simulink model "ROS_SIMULINK_Concept_Testing_ABB_6DOF"  (R2023a)
settings: Solver=FixedStepDiscrete  StartTime=0.0  StopTime=inf  FixedStep=0.004  RelTol=1e-3
model workspace (MAT data in the model file):
  SL_ROS_VariableLengthArrays_MaxSizes.CommonInfo.ArrayTruncateAction = 'EmitWarning'
  SL_ROS_VariableLengthArrays_MaxSizes.MsgTypeMap = containers.Map
  SL_ROS_VariableLengthArrays_MaxSizes.MsgTypeMap.serialization.keys = {'std_msgs/Float64MultiArray'}
  SL_ROS_VariableLengthArrays_MaxSizes.MsgTypeMap.serialization.values{1}.PropertyName = 'Data'
  SL_ROS_VariableLengthArrays_MaxSizes.MsgTypeMap.serialization.values{1}.DataType = 'double'
  SL_ROS_VariableLengthArrays_MaxSizes.MsgTypeMap.serialization.values{1}.MaxLength = 6
  SL_ROS_VariableLengthArrays_MaxSizes.MsgTypeMap.serialization.uniformity = 0
  SL_ROS_VariableLengthArrays_MaxSizes.MsgTypeMap.serialization.keyType = 'char'
  SL_ROS_VariableLengthArrays_MaxSizes.MsgTypeMap.serialization.valueType = 'any'
undefined symbols (not defined in the file): Data, Data_SL_Info
libraries: slpidlib x6, robotlib x3, simulink x3, eeGeneralControl x2, simulink_extras x1
settings Model: Creator=LYA31  LastModifiedBy=LYA31
settings OptimizationCC: EnhancedBackFolding=on  PassReuseOutputArgsAs=Individual arguments  ZeroExternalMemoryAtStartup=off  ZeroInternalMemoryAtStartup=off  MaxStackSize=64  OptimizeBlockOrder=speed  DifferentSizesBufferReuse=on  EfficientTunableParamExpr=on
settings DebuggingCC: ParameterTunabilityLossMsg=error
settings HardwareCC: ProdBitPerPointer=32  ProdBitPerSizeT=32  ProdBitPerPtrDiffT=32  ProdLargestAtomicFloat=None  ProdIntDivRoundTo=Undefined  ProdEndianess=Unspecified  ProdWordSize=32  ProdHWDeviceType=Generic->Unspecified (assume 32-bit Generic)
settings SFSimCC: MATLABDynamicMemAlloc=off
settings RTWCC: Description=Embedded Coder  SystemTargetFile=ert.tlc  HardwareBoard=Robot Operating System (ROS)  TLCOptions="-aInlineSetEventsForThisBaseRateFcn=TLC_FALSE -aSuppressMultiTaskScheduler=TLC_FALSE  -aRateBasedStepFcn=0"  TemplateMakefile=ert_default_tmf  Toolchain=Catkin  TargetLang=C++
settings CodeAppCC: ForceParamTrailComments=on  IgnoreCustomStorageClasses=off  OperatorAnnotations=on  SimulinkDataObjDesc=on  SFDataObjDesc=on  InsertBlockDesc=on

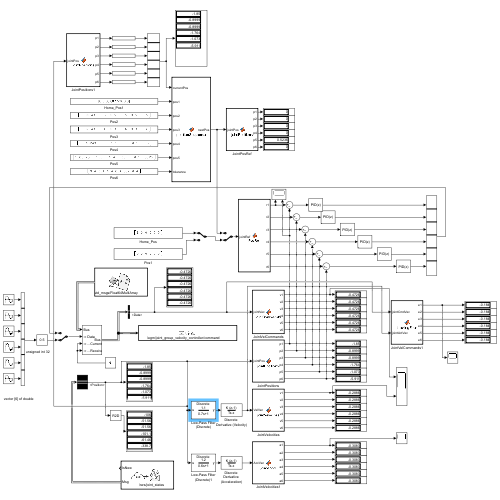
[thumbnail: Simulink's stored preview of the top-level diagram]
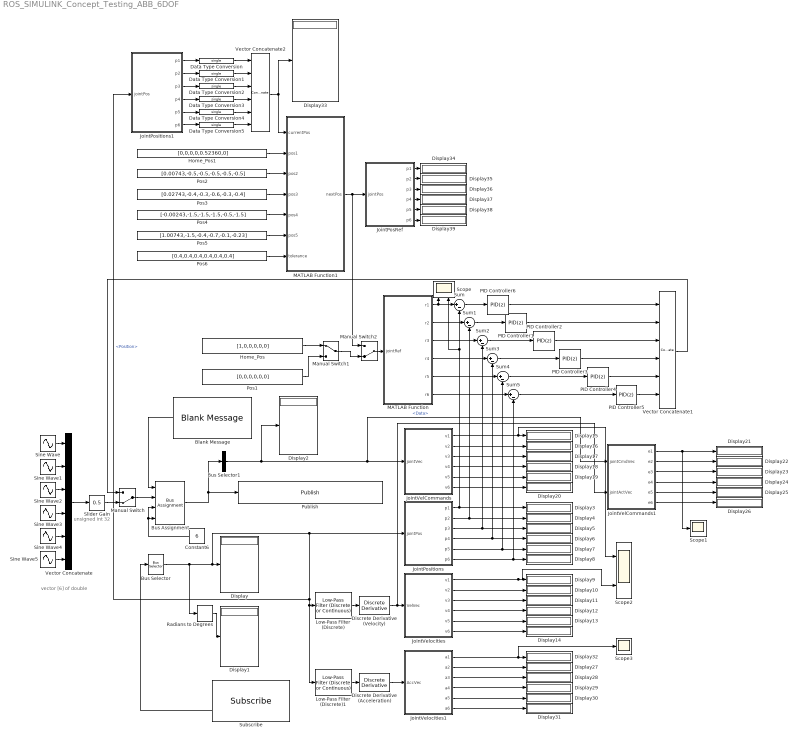
== system ROS_SIMULINK_Concept_Testing_ABB_6DOF ==
  note: unsigned int 32
  note: vector [6] of double
  Blank Message : robotlib/Blank Message  messageClass=Message  entityType=std_msgs/Float64MultiArray  messageType=std_msgs/Float64MultiArray  SampleTime=inf  legacyBusStruct=off
  Bus Assignment : BusAssignment  AssignedSignals=Data,Data_SL_Info.CurrentLength,Data_SL_Info.ReceivedLength
  Bus Selector : BusSelector  OutputSignals=Position
  Bus Selector1 : BusSelector  OutputSignals=Data
  Constant6 : Constant  Value=6  OutDataTypeStr=uint32  SampleTime=0.004
  Data Type Conversion{,1..5} (6 alike) : DataTypeConversion  OutDataTypeStr=single  SaturateOnIntegerOverflow=off  RndMeth=Floor
  Discrete Derivative (Acceleration) : simulink/Discrete/Discrete Derivative  gainval=1.0  ICPrevScaledInput=0.0  OutMin=[]  OutMax=[]  OutDataTypeStr=double  OutputDataTypeScalingMode=double  OutDataType=fixdt(1, 16)  OutScaling=2^-10  DoSatur=off
  Discrete Derivative (Velocity) : simulink/Discrete/Discrete Derivative  gainval=1.0  ICPrevScaledInput=0.0  OutMin=[]  OutMax=[]  OutDataTypeStr=double  OutputDataTypeScalingMode=double  OutDataType=fixdt(1, 16)  OutScaling=2^-10  DoSatur=off
  Display{,1..39} (40 alike) : Display
  Home_Pos : Constant  Value=[1,0,0,0,0,0]
  Home_Pos1 : Constant  Value=[0,0,0,0,0.52360,0]  OutDataTypeStr=double
  JointPosRef : MATLAB Function  TreatAsAtomicUnit=on
  JointPositions : MATLAB Function  TreatAsAtomicUnit=on
  JointPositions1 : MATLAB Function  TreatAsAtomicUnit=on
  JointVelCommands : MATLAB Function  TreatAsAtomicUnit=on
  JointVelCommands1 : MATLAB Function  TreatAsAtomicUnit=on
  JointVelocities : MATLAB Function  TreatAsAtomicUnit=on
  JointVelocities1 : MATLAB Function  TreatAsAtomicUnit=on
  Low-Pass Filter (Discrete) : eeGeneralControl/Low-Pass Filter (Discrete or Continuous)  K=1.1  T=0.7  B=inf  A=-inf  init_option=Inherited from block input  x0=0  Ts=-1
  Low-Pass Filter (Discrete)1 : eeGeneralControl/Low-Pass Filter (Discrete or Continuous)  K=1.2  T=0.6  B=inf  A=-inf  init_option=Inherited from block input  x0=0  Ts=-1
  MATLAB Function : MATLAB Function  TreatAsAtomicUnit=on
  MATLAB Function1 : MATLAB Function  TreatAsAtomicUnit=on
  Manual Switch : ManualSwitch  CurrentSetting=0
  Manual Switch1 : ManualSwitch
  Manual Switch2 : ManualSwitch  CurrentSetting=0
  PID Controller{1..5} (5 alike) : slpidlib/PID Controller  Controller=PID  Form=Ideal  TimeDomain=Discrete-time  UseExternalTs=off  SampleTime=-1  IntegratorMethod=Forward Euler  FilterMethod=Forward Euler  ControllerParametersSource=internal  P=2.4  I=0.01  UseKiTs=off  D=0.7  N=100  UseFilter=on  TunerSelectOption=Transfer Function Based (PID Tuner App)  InitialConditionSource=internal  InitialConditionForIntegrator=0  InitialConditionForFilter=0  DifferentiatorICPrevScaledInput=0  ExternalReset=none  TrackingMode=off  Kt=1  LimitOutput=off  SatLimitsSource=internal  UpperSaturationLimit=inf  LowerSaturationLimit=-inf  LinearizeAsGain=on  AntiWindupMode=none  Kb=1  LimitIntegrator=off  UpperIntegratorSaturationLimit=inf  LowerIntegratorSaturationLimit=-inf  POutMin=[]  POutMax=[]  IOutMin=[]  IOutMax=[]  DOutMin=[]  DOutMax=[]  NOutMin=[]  NOutMax=[]  SumOutMin=[]  SumOutMax=[]  SaturationOutMin=[]  SaturationOutMax=[]  PParamMin=[]  PParamMax=[]  IParamMin=[]  IParamMax=[]  DParamMin=[]  DParamMax=[]  NParamMin=[]  NParamMax=[]  KbParamMin=[]  KbParamMax=[]  KtParamMin=[]  KtParamMax=[]  KbOutMin=[]  KbOutMax=[]  KtOutMin=[]  KtOutMax=[]  IntegratorOutMin=[]  IntegratorOutMax=[]  FilterOutMin=[]  FilterOutMax=[]  SumI1OutMin=[]  SumI1OutMax=[]  SumI2OutMin=[]  SumI2OutMax=[]  SumI3OutMin=[]  SumI3OutMax=[]  SumI4OutMin=[]  SumI4OutMax=[]  SumDOutMin=[]  SumDOutMax=[]  DifferentiatorOutMin=[]  DifferentiatorOutMax=[]  FilterDiffOutCoefMin=[]  FilterDiffOutCoefMax=[]  ReciprocalOutMin=[]  ReciprocalOutMax=[]  SumDenOutMin=[]  SumDenOutMax=[]  SumNumOutMin=[]  SumNumOutMax=[]  DivideOutMin=[]  DivideOutMax=[]  UdiffTsProdOutMin=[]  UdiffTsProdOutMax=[]  NTsProdOutMin=[]  NTsProdOutMax=[]  UintegralTsProdOutMin=[]  UintegralTsProdOutMax=[]  UngainTsProdOutMin=[]  UngainTsProdOutMax=[]  ClampingZeroOutDataTypeStr=Inherit: Inherit via back propagation  ClampingZeroOutMin=[]  ClampingZeroOutMax=[]  FilterDenConstantOutDataTypeStr=Inherit: Inherit via back propagation  FilterDenConstantOutMin=[]  FilterDenConstantOutMax=[]  PCopyOutDataTypeStr=Inherit: Inherit via back propagation  PCopyOutMin=[]  PCopyOutMax=[]  NCopyOutDataTypeStr=Inherit: Inherit via back propagation  NCopyOutMin=[]  NCopyOutMax=[]  IntegratorContinuousStateAttributes=''  IntegratorStateMustResolveToSignalObject=off  IntegratorRTWStateStorageClass=Auto  FilterContinuousStateAttributes=''  FilterStateMustResolveToSignalObject=off  FilterRTWStateStorageClass=Auto  ParallelPVariant=Passthrough  IdealPVariant=InternalParameters  IVariant=InternalParameters  DVariant=InternalParameters  IntegratorVariant=Discrete  SatVariant=Disabled  AWVariant=Passthrough  PCopyVariant=Disabled  TRVariant=Disabled  FdbkBlocksVariant=Forward  IdealPFdbkVariant=Disabled  SatFdbkVariant=Disabled  DerivativeFilterVariant=ForwardEulerFilter  NVariant=InternalParameters  NCopyVariant=Disabled  FilterICVariant=InternalICsFilter  IntegratorICVariant=InternalICs  ExternalResetVariant=Disabled  TRSumVariant=Passthrough  SumFdbkVariant=Disabled  SumVariant=Sum_PID  TsampFilterVariant=InternalTs  TsampNgainVariant=Passthrough  TsampIntegralVariant=Disabled_SignalSpec  ExternalSaturationOutDataTypeStr=Inherit: Same as second input
  PID Controller6 : slpidlib/PID Controller  Controller=PID  Form=Ideal  TimeDomain=Discrete-time  UseExternalTs=off  SampleTime=-1  IntegratorMethod=Forward Euler  FilterMethod=Forward Euler  ControllerParametersSource=internal  P=9  I=0  UseKiTs=off  D=0  N=100  UseFilter=on  TunerSelectOption=Transfer Function Based (PID Tuner App)  InitialConditionSource=internal  InitialConditionForIntegrator=0  InitialConditionForFilter=0  DifferentiatorICPrevScaledInput=0  ExternalReset=none  TrackingMode=off  Kt=1  LimitOutput=off  SatLimitsSource=internal  UpperSaturationLimit=inf  LowerSaturationLimit=-inf  LinearizeAsGain=on  AntiWindupMode=none  Kb=1  LimitIntegrator=off  UpperIntegratorSaturationLimit=inf  LowerIntegratorSaturationLimit=-inf  POutMin=[]  POutMax=[]  IOutMin=[]  IOutMax=[]  DOutMin=[]  DOutMax=[]  NOutMin=[]  NOutMax=[]  SumOutMin=[]  SumOutMax=[]  SaturationOutMin=[]  SaturationOutMax=[]  PParamMin=[]  PParamMax=[]  IParamMin=[]  IParamMax=[]  DParamMin=[]  DParamMax=[]  NParamMin=[]  NParamMax=[]  KbParamMin=[]  KbParamMax=[]  KtParamMin=[]  KtParamMax=[]  KbOutMin=[]  KbOutMax=[]  KtOutMin=[]  KtOutMax=[]  IntegratorOutMin=[]  IntegratorOutMax=[]  FilterOutMin=[]  FilterOutMax=[]  SumI1OutMin=[]  SumI1OutMax=[]  SumI2OutMin=[]  SumI2OutMax=[]  SumI3OutMin=[]  SumI3OutMax=[]  SumI4OutMin=[]  SumI4OutMax=[]  SumDOutMin=[]  SumDOutMax=[]  DifferentiatorOutMin=[]  DifferentiatorOutMax=[]  FilterDiffOutCoefMin=[]  FilterDiffOutCoefMax=[]  ReciprocalOutMin=[]  ReciprocalOutMax=[]  SumDenOutMin=[]  SumDenOutMax=[]  SumNumOutMin=[]  SumNumOutMax=[]  DivideOutMin=[]  DivideOutMax=[]  UdiffTsProdOutMin=[]  UdiffTsProdOutMax=[]  NTsProdOutMin=[]  NTsProdOutMax=[]  UintegralTsProdOutMin=[]  UintegralTsProdOutMax=[]  UngainTsProdOutMin=[]  UngainTsProdOutMax=[]  ClampingZeroOutDataTypeStr=Inherit: Inherit via back propagation  ClampingZeroOutMin=[]  ClampingZeroOutMax=[]  FilterDenConstantOutDataTypeStr=Inherit: Inherit via back propagation  FilterDenConstantOutMin=[]  FilterDenConstantOutMax=[]  PCopyOutDataTypeStr=Inherit: Inherit via back propagation  PCopyOutMin=[]  PCopyOutMax=[]  NCopyOutDataTypeStr=Inherit: Inherit via back propagation  NCopyOutMin=[]  NCopyOutMax=[]  IntegratorContinuousStateAttributes=''  IntegratorStateMustResolveToSignalObject=off  IntegratorRTWStateStorageClass=Auto  FilterContinuousStateAttributes=''  FilterStateMustResolveToSignalObject=off  FilterRTWStateStorageClass=Auto  ParallelPVariant=Passthrough  IdealPVariant=InternalParameters  IVariant=InternalParameters  DVariant=InternalParameters  IntegratorVariant=Discrete  SatVariant=Disabled  AWVariant=Passthrough  PCopyVariant=Disabled  TRVariant=Disabled  FdbkBlocksVariant=Forward  IdealPFdbkVariant=Disabled  SatFdbkVariant=Disabled  DerivativeFilterVariant=ForwardEulerFilter  NVariant=InternalParameters  NCopyVariant=Disabled  FilterICVariant=InternalICsFilter  IntegratorICVariant=InternalICs  ExternalResetVariant=Disabled  TRSumVariant=Passthrough  SumFdbkVariant=Disabled  SumVariant=Sum_PID  TsampFilterVariant=InternalTs  TsampNgainVariant=Passthrough  TsampIntegralVariant=Disabled_SignalSpec  ExternalSaturationOutDataTypeStr=Inherit: Same as second input
  Pos1 : Constant  Value=[0,0,0,0,0,0]
  Pos2 : Constant  Value=[0.00743,-0.5,-0.5,-0.5,-0.5,-0.5]  OutDataTypeStr=double
  Pos3 : Constant  Value=[0.02743,-0.4,-0.3,-0.6,-0.3,-0.4]  OutDataTypeStr=double
  Pos4 : Constant  Value=[-0.00243,-1.5,-1.5,-1.5,-0.5,-1.5]  OutDataTypeStr=double
  Pos5 : Constant  Value=[1.00743,-1.5,-0.4,-0.7,-0.1,-0.23]  OutDataTypeStr=double
  Pos6 : Constant  Value=[0.4,0.4,0.4,0.4,0.4,0.4]  OutDataTypeStr=double
  Publish : robotlib/Publish  topicSource=Select from ROS network  topic=/egm/joint_group_velocity_controller/command  messageType=std_msgs/Float64MultiArray  legacyBusStruct=off  messageQueueLength=1
  Radians to Degrees : simulink_extras/Transformations/Radians to Degrees
  Scope : Scope  NumInputPorts=2
  Scope1 : Scope
  Scope2 : Scope  NumInputPorts=2
  Scope3 : Scope
  Sine Wave{,1..5} (6 alike) : Sin  Frequency=0.5  SampleTime=0.004
  Slider Gain : simulink/Math Operations/Slider Gain  gain=0.5  low=-6  high=6
  Subscribe : robotlib/Subscribe  topicSource=Select from ROS network  topic=/rws/joint_states  messageType=sensor_msgs/JointState  SampleTime=-1  legacyBusStruct=off  messageQueueLength=1
  Sum{,1..5} (6 alike) : Sum  Inputs=|+-
  Vector Concatenate : Concatenate  NumInputs=6
  Vector Concatenate1 : Concatenate  NumInputs=6
  Vector Concatenate2 : Concatenate  NumInputs=6
  wires:
  Subscribe/2 -> Bus Selector/1
  Bus Selector/1 -> Radians to Degrees/1, JointPositions1/1(jointPos), Low-Pass Filter (Discrete)1/1, Low-Pass Filter (Discrete)/1, JointPositions/1(jointPos), Display/1  "<Position>"
  Radians to Degrees/1 -> Display1/1
  Bus Assignment/1 -> Publish/1, Bus Selector1/1
  Blank Message/1 -> Bus Assignment/1
  Bus Selector1/1 -> Display2/1, JointVelCommands/1(jointVec), JointVelCommands1/1(jointCmdVec)  "<Data>"
  Vector Concatenate/1 -> Slider Gain/1
  Constant6/1 -> Bus Assignment/3, Bus Assignment/4
  JointPositions/2(p2) -> Display4/1, Sum1/2
  JointPositions/3(p3) -> Display5/1, Sum2/2
  JointPositions/4(p4) -> Display6/1, Sum3/2
  JointPositions/5(p5) -> Display7/1, Sum4/2
  JointPositions/6(p6) -> Sum5/2, Display8/1
  Sine Wave/1 -> Vector Concatenate/1
  Sine Wave1/1 -> Vector Concatenate/2
  Sine Wave2/1 -> Vector Concatenate/3
  Sine Wave3/1 -> Vector Concatenate/4
  Sine Wave4/1 -> Vector Concatenate/5
  Sine Wave5/1 -> Vector Concatenate/6
  JointPositions/1(p1) -> Scope/2, Sum/2, Display3/1
  Low-Pass Filter (Discrete)/1 -> Discrete Derivative (Velocity)/1
  JointVelocities/2(v2) -> Display10/1
  JointVelocities/5(v5) -> Display13/1
  JointVelocities/1(v1) -> Scope2/2, Display9/1
  JointVelocities/6(v6) -> Display14/1
  JointVelocities/3(v3) -> Display11/1
  JointVelocities/4(v4) -> Display12/1
  JointVelCommands/2(v2) -> Display16/1
  JointVelCommands/5(v5) -> Display19/1
  JointVelCommands/1(v1) -> Scope2/1, Display15/1
  JointVelCommands/6(v6) -> Display20/1
  JointVelCommands/3(v3) -> Display17/1
  JointVelCommands/4(v4) -> Display18/1
  JointVelCommands1/5(e5) -> Display25/1
  JointVelCommands1/1(e1) -> Scope1/1, Display21/1
  JointVelCommands1/6(e6) -> Display26/1
  JointVelCommands1/2(e2) -> Display22/1
  JointVelCommands1/4(e4) -> Display24/1
  JointVelCommands1/3(e3) -> Display23/1
  Discrete Derivative (Acceleration)/1 -> JointVelocities1/1(AccVec)
  Low-Pass Filter (Discrete)1/1 -> Discrete Derivative (Acceleration)/1
  JointVelocities1/6(a6) -> Display31/1
  JointVelocities1/1(a1) -> Scope3/1, Display32/1
  JointVelocities1/3(a3) -> Display28/1
  JointVelocities1/4(a4) -> Display29/1
  JointVelocities1/5(a5) -> Display30/1
  JointVelocities1/2(a2) -> Display27/1
  Manual Switch/1 -> Bus Assignment/2
  Slider Gain/1 -> Manual Switch/2
  MATLAB Function/1(r1) -> Sum/1, Scope/1
  MATLAB Function/2(r2) -> Sum1/1
  MATLAB Function/3(r3) -> Sum2/1
  MATLAB Function/4(r4) -> Sum3/1
  MATLAB Function/5(r5) -> Sum4/1
  MATLAB Function/6(r6) -> Sum5/1
  Sum/1 -> PID Controller6/1
  Sum1/1 -> PID Controller1/1
  Sum2/1 -> PID Controller2/1
  Sum3/1 -> PID Controller3/1
  Sum4/1 -> PID Controller4/1
  Sum5/1 -> PID Controller5/1
  PID Controller6/1 -> Vector Concatenate1/1
  PID Controller1/1 -> Vector Concatenate1/2
  PID Controller2/1 -> Vector Concatenate1/3
  PID Controller3/1 -> Vector Concatenate1/4
  PID Controller4/1 -> Vector Concatenate1/5
  PID Controller5/1 -> Vector Concatenate1/6
  Vector Concatenate1/1 -> Manual Switch/1
  Home_Pos/1 -> Manual Switch1/1
  Pos1/1 -> Manual Switch1/2
  Manual Switch1/1 -> Manual Switch2/2
  Manual Switch2/1 -> MATLAB Function/1(jointRef)
  MATLAB Function1/1(nextPos) -> JointPosRef/1(jointPos), Manual Switch2/1
  Home_Pos1/1 -> MATLAB Function1/2(pos1)
  Pos2/1 -> MATLAB Function1/3(pos2)
  Pos3/1 -> MATLAB Function1/4(pos3)
  Pos4/1 -> MATLAB Function1/5(pos4)
  Pos5/1 -> MATLAB Function1/6(pos5)
  Pos6/1 -> MATLAB Function1/7(tolerance)
  JointPositions1/1(p1) -> Data Type Conversion/1
  JointPositions1/2(p2) -> Data Type Conversion1/1
  JointPositions1/3(p3) -> Data Type Conversion2/1
  JointPositions1/4(p4) -> Data Type Conversion3/1
  JointPositions1/5(p5) -> Data Type Conversion4/1
  JointPositions1/6(p6) -> Data Type Conversion5/1
  Vector Concatenate2/1 -> Display33/1, MATLAB Function1/1(currentPos)
  Data Type Conversion/1 -> Vector Concatenate2/1
  Data Type Conversion1/1 -> Vector Concatenate2/2
  Data Type Conversion2/1 -> Vector Concatenate2/3
  Data Type Conversion3/1 -> Vector Concatenate2/4
  Data Type Conversion4/1 -> Vector Concatenate2/5
  Data Type Conversion5/1 -> Vector Concatenate2/6
  JointPosRef/2(p2) -> Display35/1
  JointPosRef/1(p1) -> Display34/1
  JointPosRef/3(p3) -> Display36/1
  JointPosRef/4(p4) -> Display37/1
  JointPosRef/5(p5) -> Display38/1
  JointPosRef/6(p6) -> Display39/1
  Discrete Derivative (Velocity)/1 -> JointVelocities/1(VelVec), JointVelCommands1/2(jointActVec)

== matlab function ROS_SIMULINK_Concept_Testing_ABB_6DOF/JointPosRef ==
  data: jointPos input; p1 output; p2 output; p3 output; p4 output; p5 output; p6 output
function [p1, p2, p3, p4, p5, p6] = jointPositions(jointPos)
    % Unpack each joint position from the vector
    p1 = jointPos(1);
    p2 = jointPos(2);
    p3 = jointPos(3);
    p4 = jointPos(4);
    p5 = jointPos(5);
    p6 = jointPos(6);
end

== matlab function ROS_SIMULINK_Concept_Testing_ABB_6DOF/JointVelCommands ==
  data: jointVec input; v1 output; v2 output; v3 output; v4 output; v5 output; v6 output
function [v1, v2, v3, v4, v5, v6] = jointCommands(jointVec)
    % Unpack each joint position from the vector
    v1 = jointVec(1);
    v2 = jointVec(2);
    v3 = jointVec(3);
    v4 = jointVec(4);
    v5 = jointVec(5);
    v6 = jointVec(6);
end

== matlab function ROS_SIMULINK_Concept_Testing_ABB_6DOF/JointPositions ==
  data: jointPos input; p1 output; p2 output; p3 output; p4 output; p5 output; p6 output
function [p1, p2, p3, p4, p5, p6] = jointPositions(jointPos)
    % Unpack each joint position from the vector
    p1 = jointPos(1);
    p2 = jointPos(2);
    p3 = jointPos(3);
    p4 = jointPos(4);
    p5 = jointPos(5);
    p6 = jointPos(6);
end

== matlab function ROS_SIMULINK_Concept_Testing_ABB_6DOF/JointVelocities ==
  data: VelVec input; v1 output; v2 output; v3 output; v4 output; v5 output; v6 output
function [v1, v2, v3, v4, v5, v6] = jointVelocities(VelVec)
    % Unpack each joint position from the vector
    v1 = VelVec(1);
    v2 = VelVec(2);
    v3 = VelVec(3);
    v4 = VelVec(4);
    v5 = VelVec(5);
    v6 = VelVec(6);
end

== matlab function ROS_SIMULINK_Concept_Testing_ABB_6DOF/JointVelCommands1 ==
  data: jointCmdVec input; e1 output; e2 output; e3 output; e4 output; e5 output; e6 output; jointActVec input
function [e1, e2, e3, e4, e5, e6] = trackingError(jointCmdVec, jointActVec)
    % Calculate the tracking error for each joint
    e1 = jointCmdVec(1) - jointActVec(1);
    e2 = jointCmdVec(2) - jointActVec(2);
    e3 = jointCmdVec(3) - jointActVec(3);
    e4 = jointCmdVec(4) - jointActVec(4);
    e5 = jointCmdVec(5) - jointActVec(5);
    e6 = jointCmdVec(6) - jointActVec(6);
end

== matlab function ROS_SIMULINK_Concept_Testing_ABB_6DOF/JointVelocities1 ==
  data: AccVec input; a1 output; a2 output; a3 output; a4 output; a5 output; a6 output
function [a1, a2, a3, a4, a5, a6] = jointAccel(AccVec)
    % Unpack each joint position from the vector
    a1 = AccVec(1);
    a2 = AccVec(2);
    a3 = AccVec(3);
    a4 = AccVec(4);
    a5 = AccVec(5);
    a6 = AccVec(6);
end

== matlab function ROS_SIMULINK_Concept_Testing_ABB_6DOF/MATLAB Function ==
  data: jointRef input; r1 output; r2 output; r3 output; r4 output; r5 output; r6 output
function [r1, r2, r3, r4, r5, r6] = PosRef(jointRef)
    % Unpack each joint position from the vector
    r1 = jointRef(1);
    r2 = jointRef(2);
    r3 = jointRef(3);
    r4 = jointRef(4);
    r5 = jointRef(5);
    r6 = jointRef(6);
end

== matlab function ROS_SIMULINK_Concept_Testing_ABB_6DOF/MATLAB Function1 ==
  data: currentPos input; nextPos output; pos1 input; pos2 input; pos3 input; pos4 input; pos5 input; tolerance input
function nextPos = positionSequence(currentPos, pos1, pos2, pos3, pos4, pos5, tolerance)
    %#codegen

    % Define a static variable to remember the last position index
    persistent lastPosIndex;
    if isempty(lastPosIndex)
        lastPosIndex = 1; % Start with the first position
    end
    
    % Initialize nextPos with the correct size
    nextPos = zeros(6, 1);
    
    % Define the sequence of positions
    positions = [pos1(:)'; pos2(:)'; pos3(:)'; pos4(:)'; pos5(:)'];
    
    % Check if current position is within the tolerance of the target position
    targetPos = positions(lastPosIndex, :);
    if all(abs(currentPos - targetPos') <= tolerance)
        % Move to the next position if the current one is achieved
        lastPosIndex = lastPosIndex + 1;
        if lastPosIndex > size(positions, 1)
            lastPosIndex = 1;
        end
    end
    
    % Output the next target position
    nextPos = positions(lastPosIndex, :)';
end

== matlab function ROS_SIMULINK_Concept_Testing_ABB_6DOF/JointPositions1 ==
  data: jointPos input; p1 output; p2 output; p3 output; p4 output; p5 output; p6 output
function [p1, p2, p3, p4, p5, p6] = jointPositions(jointPos)
    % Unpack each joint position from the vector
    p1 = jointPos(1);
    p2 = jointPos(2);
    p3 = jointPos(3);
    p4 = jointPos(4);
    p5 = jointPos(5);
    p6 = jointPos(6);
end
